simulink model "LaneTracking"  (R2023b)
settings: Solver=ode4  StartTime=0.0  StopTime=Te  FixedStep=Ts  RelTol=1e-3
undefined symbols (not defined in the file): driving, egoCarID, targetSpeed, Ts
libraries: drivingscenarioandsensors x7, slpidlib x2, robotcorelib x2, sensorinslib x1
(part 3 of 3)

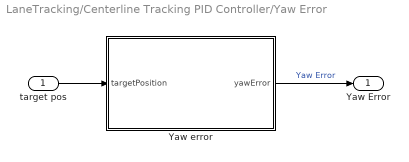
== system LaneTracking/Centerline Tracking PID Controller/Yaw Error ==
  target pos : Inport  Unit=m
  Yaw error : MATLAB Function  TreatAsAtomicUnit=on
  Yaw Error : Outport  Unit=deg
  wires:
  Yaw error/1(yawError) -> Yaw Error/1  "Yaw Error"
  target pos/1 -> Yaw error/1(targetPosition)

== matlab function LaneTracking/Lane Boundaries to centerline/calculate lane centerline  ==
  settings: sampleTime=Ts
  data: curvatureLeft input; centerlineWaypoints output size=[300, 2]; curvelengthLeft input; headingangleLeft input; lateraloffsetLeft input; curvatureRight input; curvelengthRight input; headingangleRight input; lateraloffsetRight input; Ts input; currentSpeed input
function centerlineWaypoints = calculateLaneCenterline(curvatureLeft, curvelengthLeft, headingangleLeft, lateraloffsetLeft, ...
    curvatureRight, curvelengthRight, headingangleRight, lateraloffsetRight, ...
    Ts, currentSpeed)

    % Calculate the average curvature, curve length, heading angle, and lateral offset
    curvature = (curvatureLeft + curvatureRight) / 2;
    curvelength = (curvelengthLeft + curvelengthRight) / 2;
    headingangle = (headingangleLeft + headingangleRight) / 2;
    lateraloffset = (lateraloffsetLeft + lateraloffsetRight) / 2;

    % Overspeed Tolerance m/s
    overspeed=2.25;

    % Estimate the optimal number of waypoints
    updateInterval = Ts;
    distancePerUpdate = (currentSpeed + overspeed) * updateInterval;
    totalDistance = sum(curvelength,'all');
    numPoints = max(10, ceil(totalDistance / distancePerUpdate)); % Ensure at least 10 points for very short curves
    numPoints = min(300, numPoints); % At most 300 points for very long curves
    
    % Preallocate array for waypoints
    centerlineWaypoints = NaN(300, 2); % [x, y] format

    % Generate waypoints along the centerline
    for i = 1:numPoints
        t = i / (numPoints - 1); % Normalized distance along the lane

        % Calculate x and y coordinates of the centerline waypoints
        x = curvelength * t * cosd(headingangle);
        y = curvelength * t * sind(headingangle) + lateraloffset;

        centerlineWaypoints(i, :) = [x, y];
    end
end

== matlab function LaneTracking/Centerline Tracking PID Controller/Find Next Waypoint ==
  data: centerline_car input; nextWaypoint output; CurrentSpeed input; Ts input
function nextWaypoint = findNextWaypoint(centerline_car, CurrentSpeed, Ts)
    % Find the first waypoint that is at least Ts ahead of the current position
    % If there is not one, then use the last waypoint
    for waypoint_index = 1:length(centerline_car)
        waypoint = centerline_car(waypoint_index,:);
        if waypoint(2) > Ts * CurrentSpeed
            break
        end
    end

    nextWaypoint = waypoint;
end

== matlab function LaneTracking/Environment/Pack Ego Actor ==
  data: pos input; a output Bus: BusActorsActors size=1; vel input; yaw input; yawRate input; ActorID input
function a = packEgo(pos,vel,yaw,yawRate,ActorID)
% Pack ego information into a single ego actor bus
%
% Imoprtant note:
% Output is a bus of type BusActorsActors. This is the same bus used by the
% Scenario Reader to output an individual actor. If you change the
% output bus name of Scenario Reader change the output bus name here
% as well by clicking on 'Edit Data' in the menu above.

a = struct(...
    'ActorID',ActorID,...
    'Position', [pos(1) pos(2) 0], ...
    'Velocity', [vel(1) vel(2) 0], ...
    'Roll', 0, ...
    'Pitch', 0, ...
    'Yaw', yaw, ...
    'AngularVelocity', [0 0 yawRate]);

== matlab function LaneTracking/Centerline Tracking PID Controller/Yaw Error/Yaw error ==
  data: yawError output; targetPosition input
function yawError= calculateYawError(targetPosition)
 
    % Calculate the desired yaw angle to face the target position
    yawError = atan2(targetPosition(2), targetPosition(1));

    % Normalize an angle to the range [-pi, pi]
    angleWrap = @(angle) mod(angle + pi, 2 * pi) - pi;
    yawError=angleWrap(yawError);

    % Prefer everything in degree
    yawError = rad2deg(yawError);
end
